simulink model "q3_simulink"  (R2023b)
settings: Solver=VariableStepAuto  StartTime=0.0  StopTime=5  RelTol=1e-3
values from neighbouring files (symbols this model uses):
  A = [0, 1,      0;       0, -b/J,   K/J;       0, -K/L, -R/L;]    [lec7_dc_motor_control_example.m]    (also in lec7_example_11.m = [0 0 4 1; lec7_notes_example_11.m = [-1, 1, 0;       0,  1, 1;       0,  0, 2;]; mini_proj_1.m = [-8.8487 + (a-b)/5,     -0.0399,              -5.55 + (c+d)/; mini_proj_q1.m = [-8.8487 + (a-b)/5,     -0.0399,              -5.55 + (c+d)/)
  B = [0;       0;       1/L;]    [lec7_dc_motor_control_example.m]    (also in lec7_example_11.m = [-2 0; lec7_notes_example_11.m = [1, 1;       0, 0;       0, 1;]; mini_proj_1.m = [0.0564+(b)/(10+c),           0.0319;       0.0165-(c+d-5)/(; mini_proj_q1.m = [0.0564+(b)/(10+c),           0.0319)
  C = [1, 0, 0]    [lec7_dc_motor_control_example.m]    (also in lec7_notes_example_11.m = [1, 3, -1;      0, 1,  0;]; mini_proj_1.m = [-3.2988,           -2.1932+(10*c+d)/(100+5*a), 0.0370,  -0.; mini_proj_q1.m = [-3.2988,           -2.1932+(10*c+d)/(100+5*a), 0.0370,  -0.; mini_proj_q2.m = [-3.2988,           -2.1932+(10*c+d)/(100+5*a), 0.0370,  -0.)
  C_T_matrix_inv = inv(C_T_matrix)    [q3_full.m]    (also in q5_full.m = [-0.292392890492903   0.278799577693527  -0.115994901359206 )
  D = [0, 0 ... (first row only)    [q1_full.m]    (also in q1_params.m; q2_full.m; q3_full.m = [-1 0; q4_full.m)
  E = T * B    [q3_full.m]    (also in q5_full.m = [-0.179108013653627  -0.106649750104643)
  G = double(subs(G, [struct('g1_1', 1, 'g1_2', 0, 'g2_1', 0, 'g2_2', 1)]))    [q3_full.m]    (also in q4_full.m = simplify(vpa(C) * vpa(inv( s*eye(n,n) - A )) * vpa(B)); q5_full.m = [1 0)
  K = transpose(place(A, B, des_poles))    [lec7_dc_motor_control_example.m]    (also in lec7_example_11.m = K_bar * T; lec7_notes_example_11.m = K_bar * T; mini_proj_1.m = K_bar * T; mini_proj_q1.m = K_bar * T)
  x_0 = [0.5; -0.1; 0.3; -0.8;]    [mini_proj_1.m]    (also in mini_proj_q1.m; mini_proj_q2.m; q1_full.m; q1_params.m)
settings Model: Creator=john  LastModifiedBy=john

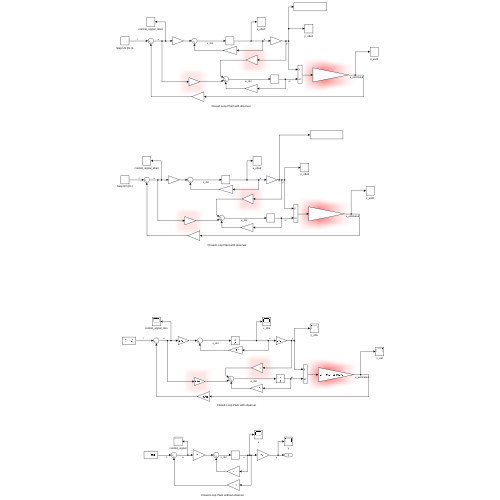
[thumbnail: Simulink's stored preview of the top-level diagram]
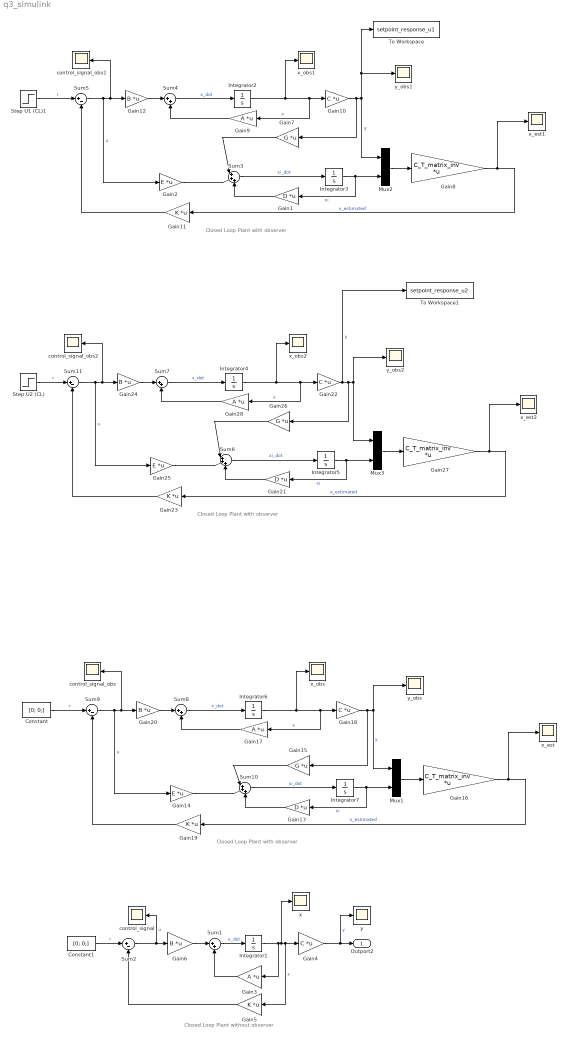
== system q3_simulink ==
  note: Closed Loop Plant with observer
  note: Closed Loop Plant without observer
  note: Closed Loop Plant with observer
  note: Closed Loop Plant with observer
  Constant : Constant  Value=[0; 0;]
  Constant1 : Constant  Value=[0; 0;]
  Gain1 : Gain  Gain=D  Multiplication=Matrix(K*u)
  Gain{4,10,18,22} (4 alike) : Gain  Gain=C  Multiplication=Matrix(K*u)
  Gain{5,11,19,23} (4 alike) : Gain  Gain=K  Multiplication=Matrix(K*u)
  Gain{6,12,20,24} (4 alike) : Gain  Gain=B  Multiplication=Matrix(K*u)
  Gain13 : Gain  Gain=D  Multiplication=Matrix(K*u)
  Gain14 : Gain  Gain=E  Multiplication=Matrix(K*u)
  Gain15 : Gain  Gain=G  Multiplication=Matrix(K*u)
  Gain16 : Gain  Gain=C_T_matrix_inv  Multiplication=Matrix(K*u)
  Gain{3,9,17,28} (4 alike) : Gain  Gain=A  Multiplication=Matrix(K*u)
  Gain2 : Gain  Gain=E  Multiplication=Matrix(K*u)
  Gain21 : Gain  Gain=D  Multiplication=Matrix(K*u)
  Gain25 : Gain  Gain=E  Multiplication=Matrix(K*u)
  Gain26 : Gain  Gain=G  Multiplication=Matrix(K*u)
  Gain27 : Gain  Gain=C_T_matrix_inv  Multiplication=Matrix(K*u)
  Gain7 : Gain  Gain=G  Multiplication=Matrix(K*u)
  Gain8 : Gain  Gain=C_T_matrix_inv  Multiplication=Matrix(K*u)
  Integrator1 : Integrator  InitialCondition=x_0
  Integrator{2..5,7} (5 alike) : Integrator
  Integrator6 : Integrator  InitialCondition=x_0
  Mux1 : Mux  Inputs=2
      settings: DisplayOption=signals
  Mux2 : Mux  Inputs=2
      settings: DisplayOption=signals
  Mux3 : Mux  Inputs=2
      settings: DisplayOption=signals
  Step U1 (CL)1 : Step  Time=0  Before=[0; 0;];  After=[1; 0;];  SampleTime=0
  Step U2 (CL) : Step  Time=0  Before=[0; 0;];  After=[0; 1;];  SampleTime=0
  Sum{1,4,7..8} (4 alike) : Sum  Inputs=|++
  Sum10 : Sum  Inputs=|+++
  Sum{2,5,9,11} (4 alike) : Sum  Inputs=|+-
  Sum3 : Sum  Inputs=|+++
  Sum6 : Sum  Inputs=|+++
  To Workspace : ToWorkspace  VariableName=setpoint_response_u1  SaveFormat=Timeseries  SampleTime=-1
  To Workspace1 : ToWorkspace  VariableName=setpoint_response_u2  SaveFormat=Timeseries  SampleTime=-1
  control_signal : Scope
  control_signal_obs : Scope
  control_signal_obs1 : Scope
  control_signal_obs2 : Scope
  x : Scope
  x_est : Scope
  x_est1 : Scope
  x_est2 : Scope
  x_obs : Scope
  x_obs1 : Scope
  x_obs2 : Scope
  y : Scope
  y_obs : Scope
  y_obs1 : Scope
  y_obs2 : Scope
  Outport2 : Outport
  wires:
  Sum8/1 -> Integrator6/1  "x_dot"
  Gain18/1 -> y_obs/1, Mux1/1, Gain15/1  "y"
  Gain19/1 -> Sum9/2
  Sum10/1 -> Integrator7/1  "xi_dot"
  Gain15/1 -> Sum10/1
  Gain20/1 -> Sum8/1
  Mux1/1 -> Gain16/1
  Gain13/1 -> Sum10/3
  Sum9/1 -> control_signal_obs/1, Gain20/1, Gain14/1  "u"
  Gain17/1 -> Sum8/2
  Gain14/1 -> Sum10/2
  Integrator6/1 -> x_obs/1, Gain18/1, Gain17/1  "x"
  Constant/1 -> Sum9/1  "r"
  Gain16/1 -> x_est/1, Gain19/1  "x_estimated"
  Integrator7/1 -> Gain13/1, Mux1/2  "xi"
  Sum1/1 -> Integrator1/1  "x_dot"
  Sum2/1 -> control_signal/1, Gain6/1  "u"
  Gain6/1 -> Sum1/1
  Gain4/1 -> y/1, Outport2/1  "y"
  Integrator1/1 -> Gain3/1, x/1, Gain5/1, Gain4/1  "x"
  Gain5/1 -> Sum2/2
  Gain3/1 -> Sum1/2
  Constant1/1 -> Sum2/1  "r"
  Sum5/1 -> control_signal_obs1/1, Gain12/1, Gain2/1  "u"
  Integrator2/1 -> x_obs1/1, Gain10/1, Gain9/1  "x"
  Gain8/1 -> x_est1/1, Gain11/1  "x_estimated"
  Gain9/1 -> Sum4/2
  Gain2/1 -> Sum3/2
  Gain12/1 -> Sum4/1
  Integrator3/1 -> Gain1/1, Mux2/2  "xi"
  Mux2/1 -> Gain8/1
  Sum4/1 -> Integrator2/1  "x_dot"
  Gain7/1 -> Sum3/1
  Sum3/1 -> Integrator3/1  "xi_dot"
  Step U1 (CL)1/1 -> Sum5/1  "r"
  Gain11/1 -> Sum5/2
  Gain1/1 -> Sum3/3
  Gain10/1 -> To Workspace/1, y_obs1/1, Mux2/1, Gain7/1  "y"
  Gain23/1 -> Sum11/2
  Sum7/1 -> Integrator4/1  "x_dot"
  Gain25/1 -> Sum6/2
  Gain27/1 -> x_est2/1, Gain23/1  "x_estimated"
  Integrator4/1 -> x_obs2/1, Gain22/1, Gain28/1  "x"
  Integrator5/1 -> Gain21/1, Mux3/2  "xi"
  Gain21/1 -> Sum6/3
  Step U2 (CL)/1 -> Sum11/1  "r"
  Gain26/1 -> Sum6/1
  Mux3/1 -> Gain27/1
  Sum11/1 -> control_signal_obs2/1, Gain24/1, Gain25/1  "u"
  Gain28/1 -> Sum7/2
  Gain22/1 -> To Workspace1/1, y_obs2/1, Mux3/1, Gain26/1  "y"
  Sum6/1 -> Integrator5/1  "xi_dot"
  Gain24/1 -> Sum7/1
